simulink library "mlepLibrary"  (R2018a)
settings: Solver=ode45  StartTime=0.0  StopTime=10.0  RelTol=1e-3
undefined symbols (not defined in the file or in its folder): cs_val, mlepBlk_callback
settings Model: Creator=willyg  LastModifiedBy=E592090
settings DataIOCC: LimitDataPoints=on  SaveFormat=Array  SignalLoggingSaveFormat=ModelDataLogs
settings OptimizationCC: BlockReduction=off  BooleanDataType=off  LifeSpan=inf
settings DebuggingCC: SaveWithParameterizedLinksMsg=none  UnderspecifiedInitializationDetection=Classic  MergeDetectMultiDrivingBlocksExec=none  SignalResolutionControl=TryResolveAllWithWarning  MultiTaskDSMMsg=warning  MultiTaskCondExecSysMsg=none  SFUnexpectedBacktrackingDiag=warning  SFNoUnconditionalDefaultTransitionDiag=warning  SFExecutionAtInitializationDiag=none
settings HardwareCC: ProdBitPerPointer=32  ProdBitPerSizeT=32  ProdBitPerPtrDiffT=32  ProdLargestAtomicFloat=None  ProdIntDivRoundTo=Undefined  ProdEndianess=Unspecified  ProdWordSize=32  ProdHWDeviceType=32-bit Generic  TargetUnknown=on
settings ModelReferenceCC: PropagateSignalLabelsOutOfModel=off
settings CodeAppCC: StateflowObjectComments=on
settings GRTTargetCC: TargetLangStandard=C89/C90 (ANSI)  GeneratePreprocessorConditionals=Disable all
settings ConfigComp: CovMetricSettings=dw  CovHtmlReporting=on  CovSaveCumulativeToWorkspaceVar=on  CovSaveSingleToWorkspaceVar=on  CovExternalEMLEnable=off

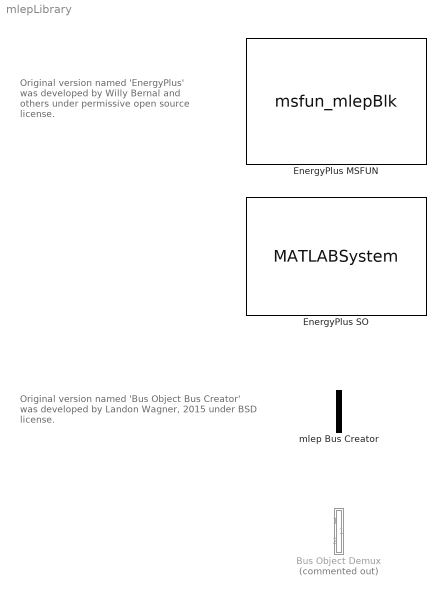
== system mlepLibrary ==
  note: Original version named 'EnergyPlus'
      | was developed by Willy Bernal and
      | others under permissive open source
      | license.
  note: Original version named 'Bus Object Bus Creator'
      | was developed by Landon Wagner, 2015 under
      | BSD license.
  Bus Object Demux : Subsystem  Commented=on  mask{busType=Bus: epInbus, bs_done=[]}
      mask prompts: busType "Bus Type"
      mask TypeOptions busType: Bus: epInbus | Bus: epOutbus
      mask Callback busType:
      | % Using variable names terminated with "_BOBC" to lessen the chances of
      | % collisions with existing workspace variables.
      | 
      | % Get the current block handle and mask handle.
      | handleCreator_BOBC = gcbh;
      | maskObj_BOBC       = Simulink.Mask.get(gcb);
      | 
      | % Get a list of variables in the workspace in order to search for the '1x1
      | % Bus' types.
      | wsVars_BOBC = whos;
      | 
      | % Reset the 'TypeOptions' bus list in case some '1x1 Bus' types have been
      | % deleted from or added to the workspace.
      | opts = {'<empty>'};
      | 
      | % Current number of options
      | old_opts = maskObj_BOBC.Parameters.TypeOptions;
      | 
      | % Reset the bus count.
      | busCount_BOBC = 0;
      | 
      | for index_BOBC = 1:length(wsVars_BOBC)
      | 
      |    % If the variable is a bus object...
      |    if strcmp(wsVars_BOBC(index_BOBC).class, 'Simulink.Bus')
      | 
      |       busCount_BOBC = busCount_BOBC + 1;
      | 
      |       % ... add it to the TypeOptions of the mask.
      |       opts(busCount_BOBC) = {['Bus: ', wsVars_BOBC(index_BOBC).name]};
      |    end
      | end
      | 
      | if busCount_BOBC == 0
      | 
      |    % If there are NO bus objects in the workspace then provide a warning
      |    % popup...
      |    %warning('There are currently no bus objects in the workspace - you have no use for this block. Use a normal Bus Creator instead.')
      | 
      |    % ... and do nothing.
      | % elseif ~strcmp(get_param(handleCreator_BOBC, 'OutDataTypeStr'), 'Inherit: auto')
      | %
      | %    % If the currently selected bus data type ('OutDataTypeStr') is not
      | %    % 'Inherit: auto' (i.e., if we are reopening the mask.) then get the
      | %    % current 'OutDataTypeStr' and 'maskVal.' ('maskVal' is the selected
      | %    % 'TypeOptions' list member.)
      | %    outDatStr_BOBC = get_param(handleCreator_BOBC, 'OutDataTypeStr');
      | %    maskVal_BOBC   = get_param(handleCreator_BOBC, 'MaskValues');
      | %
      | %    if ~strcmp(outDatStr_BOBC, maskVal_BOBC{1})
      | %
      | %       % Upon re-opening the mask if the default 'TypeOptions' list member
      | %       % (The first one.) contained in 'maskVal' does not match the
      | %       % currently selected bus data type ('OutDataTypeStr') then set the
      | %       % 'TypeOptions' list member to the selected bus data type. (Cuts down
      | %       % on confusion to have the displayed list member match the selected
      | %       % bus data type rather than the first entry.)
      | %       set_param(handleCreator_BOBC, 'MaskValues', {outDatStr_BOBC});
      | %    end
      | end
      | 
      | if ~strcmp([old_opts{:}],[opts{:}])
      |     maskObj_BOBC.Parameters.TypeOptions = opts;
      | end
      | 
      | % Clean up the workspace.
      | clear  handleCreator_BOBC  maskObj_BOBC     wsVars_BOBC ...
      |             busCount_BOBC    index_BOBC  outDatStr_BOBC ...
      |              maskVal_BOBC          opts        old_opts
      mask DialogControl applyMOCBSelection Prompt: Select signals
      mask DialogControl applyMOCBSelection Callback: run('clbk.m');
  EnergyPlus MSFUN : M-S-Function  InitFcn=mlepBlk_callback(gcb,'InitFcn');  FunctionName=msfun_mlepBlk  Parameters=work_dir, rel_path, fname, weather_profile, nout, timeout, eplus_path, bcvtb_dir, port, host  mask(EnergyPlus Cosimulation){work_dir=, rel_path=on, fname=idf_file, weather_profile=USA_IL_Chicago-OHare.Intl.AP.725300_TMY3, time_step=900, nout=2, timeout=10, mlep_defaults=on, eplus_path=, bcvtb_dir=, port=0, host=}
      mask prompts: work_dir "MLE+ working directory (empty = current directory)"; rel_path "Relative path"; fname "IDF file name"; weather_profile "EnergyPlus weather profile"; time_step "Time step (s)"; nout "Number of real outputs"; timeout "Communication timeout (s)"; mlep_defaults "Use default MLE+ settings"; eplus_path "EnergyPlus executable path (empty = default)"; bcvtb_dir "BCVTB directory (empty = default)"; port "Socket port (0 = auto)"; host "Socket host (empty = localhost)"
      mask help: This block implements cosimulation with EnergyPlus by allowing Simulink to exchange input and output data with it. Currently, EnergyPlus only supports real data.
      settings: PreSaveFcn=mlepBlk_callback(gcb,'PreSaveFcn');
      mask Help:
      | Simulate a building model using EnergyPlus
      | 
      | <h2>Description</h2>
      | This block implements <a href="http://apps1.eere.energy.gov/buildings/energyplus/">EnergyPlus</a> cosimulation by allowing Simulink to exchange input and output data with EnergyPlus at each time step.
      | 
      | When a simulation starts, this block starts EnergyPlus in parallel. During simulation, EnergyPlus exchanges data with Simulink using the <a href="http://simulationresearch.lbl.gov/bcvtb">Building Controls Virtual Test Bed</a> (BCVTB) interface via <a href="http://mlab.seas.upenn.edu/mlep/">MLE+</a>.
      | 
      | Detailed information about the interface is available in the MLE+ manual.
      | 
      | <h2>Requirements</h2>
      | Requires <a href="http://apps1.eere.energy.gov/buildings/energyplus/">EnergyPlus</a> and <a href="http://mlab.seas.upenn.edu/mlep/">MLE+</a>. In addition, requires a properly configured EnergyPlus model file (IDF) and BCVTB configuration file; see Comments.
      | 
      | <h2>Input</h2>
      | Block input <b>input</b> is a real-valued vector of EnergyPlus inputs corresponding to the inputs listed in the BCVTB config file <code>variables.cfg</code> (in order).
      | 
      | <h2>Output</h2>
      | The block outputs are, in order:
      | <dl>
      |   <dt><b>flag</b></dt><dd>Status flag for EnergyPlus: 0 if OK, non-zero for error</dd>
      |   <dt><b>time</b></dt><dd>Current simulation time of EnergyPlus (s)</dd>
      |   <dt><b>output</b></dt><dd>Real-valued vector of EnergyPlus outputs corresponding to the outputs listed in the BCVTB config file <code>variables.cfg</code> (in order).</dd>
      | </dl>
      | 
      | <h2>Parameters</h2>
      | The block mask provides inputs for all required MLE+ configuration parameters. The mask includes two tabs. The <i>Model</i> tab provides information about the EnergyPlus model to run, and the <i>MLE+</i> provides inputs for MLE+ settings.
      | 
      | String inputs in the block mask, such as paths and file names, are not evaluated prior to passing to MLE+. Therefore, MATLAB expressions which evaluate to strings (for example, <code>[pwd '/somedir']</code>) may not be passed directly. Instead, use an initialization script to evaluate these expressions and store the evaluated strings in the block mask prior to running the simulation.
      | 
      | <h3>Model Tab</h3>
      | The <i>Model</i> tab provides inputs for the following parameters:
      | <dl>
      |   <dt><b>MLE+ working directory</b></dt>
      |     <dd>The MLE+ and EnergyPlus working directory. <i>EnergyPlus will read from and write to this directory.</i></dd>
      |   <dt><b>Relative path</b></dt>
      |     <dd>Check this box if <b>MLE+ working directory</b> is specified relative to the current MATLAB working directory. <i>Otherwise, the block will treat <b>MLE+ working directory</b> as an absolute path.</i></dd>
      |   <dt><b>IDF file name</b></dt>
      |     <dd>The EnergyPlus model file (IDF), with or without the <code>.idf</code> extension. <i>This file must be included in the <b>MLE+ working directory</b>. Do not specify an absolute path for this file!</i></dd>
      |   <dt><b>EnergyPlus weather profile</b></dt>
      |     <dd>The EnergyPlus weather file (EPW), with or without the <code>.epw</code> extension. <i>A matching weather file must be included in your EnergyPlus installation's <code>WeatherData</code> directory.</i></dd>
      |   <dt><b>Time Step</b></dt>
      |     <dd>The EnergyPlus time step (s). <i>This need not be the same as the Simulink time step.</i></dd>
      |   <dt><b>Number of Real Outputs</b></dt>
      |     <dd>The number of real outputs from EnergyPlus. <i>This number must match the number of output variables in <code>variables.cfg</code>.</i></dd>
      | </dl>
      | 
      | <h3>MLE+ Tab</h3>
      | The <i>MLE+</i> tab provides inputs for the following parameters:
      | <dl>
      |   <dt><b>Communication timeout</b></dt>
      |     <dd>Time delay (s) before communication between MLE+ and EnergyPlus times out.</dd>
      |   <dt><b>Use default MLE+ settings</b></dt>
      |     <dd>Uncheck this box to gain access to the remaining settings in the <i>MLE+</i> tab.</dd>
      |   <dt><b>EnergyPlus executable path</b></dt>
      |     <dd>The full path to the EnergyPlus executable (e.g. <code>C:\EnergyPlusV8-1-0\RunEPlus.bat</code>); leave blank to use default MLE+ setting.</dd>
      |   <dt><b>BCVTB directory</b></dt>
      |     <dd>The full path to the directory where the BCVTB library resides; leave blank to use default MLE+ setting.</dd>
      |   <dt><b>Socket port</b></dt>
      |     <dd>The port to use for communication with EnergyPlus; enter <code>0</code> to allow MLE+ to automatically select a port.</dd>
      |   <dt><b>Socket host</b></dt>
      |     <dd>The IP address of the host machine where EnergyPlus runs; leave blank to use localhost (the local computer).</dd>
      | </dl>
      | 
      | <h2>Comments</h2>
      | <ol>
      |   <li>For fixed time step simulation in Simulink, the EnergyPlus time step must be an exact multiple of the Simulink time step.</li>
      |   <li>Summary of requirements for EnergyPlus model file (<code>*.idf</code>):
      |     <ol type="a">
      | 	  <li>The EnergyPlus time step specified in the file must match the value specified in the block mask.</li>
      | 	  <li>The start date and time in EnergyPlus must correspond to the start time of the Simulink simulation (usually <i>t</i> = 0 s).</li>
      | 	  <li>The <i>ExternalInterface</i> object must be defined and assigned the name  <code>PtolemyServer</code>.</li>
      | 	  <li>The file must include <i>ExternalInterface</i> definitions all inputs specified in the BCVTB config file, and the names must match.</li>
      | 	  <li>The file must include <i>Output</i> definitions all outputs specified in the BCVTB config file, and the names must match.</li>
      | 	</ol>
      |   </li>
      |   <li>Summary of requirements for BCVTB config file (<code>variables.cfg</code>):
      |     <ol type="a">
      | 	  <li>The file be located in the MLE+ working directory specified in the block mask.</li>
      | 	  <li>Number of output variables must match the value specified in the block mask.</li>
      | 	  <li>Order of input variables must match the order of elements in the input vector in Simulink.</li>
      | 	  <li>Order of output variables must match the order of elements in the output vector in Simulink.</li>
      | 	</ol>
      |   <li>For more details regarding the implementation of MLE+, the meaning of the parameters, and creating the BCVTB configuration file, see the MLE+ <a href="http://mlab.seas.upenn.edu/mlep/">documentation</a>.</li>
      | </ol>
      | 
      | <h2>References</h2>
      | <ol>
      |   <li>W. Bernal, M. Behl, T. X. Nghiem, and R. Mangharam, "MLE+: A Tool for Integrated Design and Deployment of Energy Efficient Building Controls," 4th ACM Workshop On Embedded Sensing Systems For Energy-Efficiency In Buildings, (BuildSys '12), Toronto, Canada, 2012. Available: <a href="http://repository.upenn.edu/mlab_papers/51/">http://repository.upenn.edu/mlab_papers/51/</a></li>
      | </ol>
      mask Callback mlep_defaults: mlepBlk_callback(gcb, 'MaskConfig');
      mask DialogControl ParameterTabVar0 Prompt: Model
      mask DialogControl ParameterTabVar01 Prompt: MLE+
      mask Display:
      | image(imread('mlepBlkIcon.jpg'))
      | 
      | text(0.05,.1,'EnergyPlus\nCo-simulation');
      | % Inputs
      | c = 0.80*[1 1 1];
      | x = [0 1 1 0 0];
      | y = [0 0 1 1 0];
      | h = 0.09;
      | 
      | %color('white');
      | % x0 = 0;
      | % y0 = 0.448;
      | % w = 0.18;
      | % patch(x0 + w*x, y0 + h*y, c);
      | port_label('input', 1, 'Inputs');
      | 
      | % % Outputs
      | % w = 0.128;
      | % x0 = 1-w;
      | % y0 = 0.768;
      | % patch(x0 + w*x, y0 + h*y, c);
      | port_label('output', 1, 'Flag');
      | 
      | % w = 0.139;
      | % x0 = 1-w;
      | % y0 = 0.455;
      | % patch(x0 + w*x, y0 + h*y, c);
      | port_label('output', 2, 'Time');
      | 
      | % w = 0.215;
      | % x0 = 1-w;
      | % y0 = 0.13;
      | % patch(x0 + w*x, y0 + h*y, c);
      | port_label('output', 3, 'Outputs');
  EnergyPlus SO : MATLABSystem  System=so_mlepBlk  idfFile=in.idf  epwFile=in.epw  SimulateUsing=Code generation  useBus=on  inputBusName=epInbus  outputBusName=epOutbus
      mask Type: mlepSO
      mask Display:
      | image('mlepBlkIcon.jpg');
      | port_label('input',1,'epInbus');
      | port_label('output',1,'Flag');
      | port_label('output',2,'Time');
      | port_label('output',3,'epOutbus');
  mlep Bus Creator : BusCreator  Inputs=1  mask(BUS OBJECT Bus Creator){busType=Bus: epInbus}
      mask prompts: busType "Bus Type"
      mask help:
      | Provides users the cabability to painlessly, instantly customize bus creators of output data type 'Bus:' by selecting the bus object type from a drop down menu dynamically populated by bus objects in the workspace.
      |
      | After pressing the "Apply Selection" button signal lines into the creator are populated and named with the elements in the chosen bus saving the user from having to recall and fill out signal line names.
      |
      | NOTE that when copying a Bus Object Bus Creator from your locked Library the link to the Library is automatically broken. This saves the user from having to Unlock Links To Library (From the Library menu.), Disable Link and finally Break Link (Both from the Model menu.) for every placed instance of the block.
      settings: AttributesFormatString=%<OutDataTypeStr>  CopyFcn=set_param(gcb, 'LinkStatus', 'none')
      mask TypeOptions busType: Bus: epInbus | Bus: epOutbus
      mask Callback busType:
      | % Using variable names terminated with "_BOBC" to lessen the chances of
      | % collisions with existing workspace variables.
      | 
      | % Get the current block handle and mask handle.
      | handleCreator_BOBC = gcbh;
      | maskObj_BOBC       = Simulink.Mask.get(gcb);
      | 
      | % Get a list of variables in the workspace in order to search for the '1x1
      | % Bus' types.
      | wsVars_BOBC = whos;
      | 
      | % Reset the 'TypeOptions' bus list in case some '1x1 Bus' types have been
      | % deleted from or added to the workspace.
      | opts = {'<empty>'};
      | 
      | % Current number of options
      | old_opts = maskObj_BOBC.Parameters.TypeOptions;
      | 
      | % Reset the bus count.
      | busCount_BOBC = 0;
      | 
      | for index_BOBC = 1:length(wsVars_BOBC)
      | 
      |    % If the variable is a bus object...
      |    if strcmp(wsVars_BOBC(index_BOBC).class, 'Simulink.Bus')
      | 
      |       busCount_BOBC = busCount_BOBC + 1;
      | 
      |       % ... add it to the TypeOptions of the mask.
      |       opts(busCount_BOBC) = {['Bus: ', wsVars_BOBC(index_BOBC).name]};
      |    end
      | end
      | 
      | if busCount_BOBC == 0
      | 
      |    % If there are NO bus objects in the workspace then provide a warning
      |    % popup...
      |    warning('There are currently no bus objects in the workspace - you have no use for this block. Use a normal Bus Creator instead.')
      | 
      |    % ... and do nothing.
      | elseif ~strcmp(get_param(handleCreator_BOBC, 'OutDataTypeStr'), 'Inherit: auto')
      | 
      |    % If the currently selected bus data type ('OutDataTypeStr') is not
      |    % 'Inherit: auto' (i.e., if we are reopening the mask.) then get the
      |    % current 'OutDataTypeStr' and 'maskVal.' ('maskVal' is the selected
      |    % 'TypeOptions' list member.)
      |    outDatStr_BOBC = get_param(handleCreator_BOBC, 'OutDataTypeStr');
      |    maskVal_BOBC   = get_param(handleCreator_BOBC, 'MaskValues');
      | 
      |    if ~strcmp(outDatStr_BOBC, maskVal_BOBC{1})
      | 
      |       % Upon re-opening the mask if the default 'TypeOptions' list member
      |       % (The first one.) contained in 'maskVal' does not match the
      |       % currently selected bus data type ('OutDataTypeStr') then set the
      |       % 'TypeOptions' list member to the selected bus data type. (Cuts down
      |       % on confusion to have the displayed list member match the selected
      |       % bus data type rather than the first entry.)
      |       set_param(handleCreator_BOBC, 'MaskValues', {outDatStr_BOBC});
      |    end
      | end
      | 
      | if ~strcmp([old_opts{:}],[opts{:}])
      |     maskObj_BOBC.Parameters.TypeOptions = opts;
      | end
      | 
      | % Clean up the workspace.
      | clear  handleCreator_BOBC  maskObj_BOBC     wsVars_BOBC ...
      |             busCount_BOBC    index_BOBC  outDatStr_BOBC ...
      |              maskVal_BOBC          opts        old_opts
      mask DialogControl applyMOCBSelection Prompt: Apply Selection
      mask DialogControl applyMOCBSelection Callback:
      | % Using variable names terminated with "_BOBC" to lessen the chances of
      | % collisions with existing workspace variables.
      | 
      | % Get the current block, current block handle and mask handle.
      | currentBlock_BOBC  = gcb;
      | handleCreator_BOBC = gcbh;
      | 
      | % Get the desired bus type...
      | desiredBusType_BOBC = get_param(handleCreator_BOBC, 'busType');
      | 
      | % ... and set the 'OutDataTypeStr' to it.
      | set_param(handleCreator_BOBC, 'OutDataTypeStr', desiredBusType_BOBC);
      | 
      | %% First delete any existing lines on the port.
      | % Get the line handles.
      | lh_BOBC = get_param(handleCreator_BOBC, 'LineHandles');
      | 
      | % If any lines exist (Non- -1 line handles.), delete them and start over.
      | if max(lh_BOBC.Inport > 0)
      | 
      |    for index_BOBC = 1:length(lh_BOBC.Inport)
      | 
      |       if lh_BOBC.Inport(index_BOBC) > 0
      | 
      |          delete_line(lh_BOBC.Inport(index_BOBC))
      |       end
      |    end
      | end
      | 
      | %% Then work on adding new lines.
      | 
      | % Get the block path for 'add_line' function.
      | blockPath_BOBC = get_param(handleCreator_BOBC, 'Parent');
      | 
      | % Get the newly selected bus type ('OutDataTypeStr')...
      | mocbBusType_BOBC = get_param(currentBlock_BOBC, 'OutDataTypeStr');
      | 
      | % ... and parse off "Bus: " so the string of the desired bus contained in
      | % 'OutDataTypeStr' matches the raw workspace bus names.
      | mocbBusType_BOBC = mocbBusType_BOBC(6:end);
      | 
      | % Then evaluate the string containing the workspace bus name which will
      | % load the desired bus parameters.
      | busParams_BOBC = eval(mocbBusType_BOBC);
      | 
      | % From the parameters grab the number of lines to add.
      | numLines_BOBC = length(busParams_BOBC.Elements);
      | 
      | % Set the number of inputs of the masked bus creator to the number of lines
      | % to add.
      | set_param(handleCreator_BOBC, 'Inputs', num2str(numLines_BOBC));
      | 
      | % Set heigh
      | sz = get_param(handleCreator_BOBC, 'Position');
      | y0 = sz(2) + (sz(4)-sz(2))/2; % vertical center
      | h  = max(sz(4)-sz(2), numLines_BOBC*10); % height
      | sz = [sz(1), ...
      |       y0 - h/2, ...
      |       sz(3), ...
      |       y0 + h/2];
      | set_param(handleCreator_BOBC, 'Position', sz);
      | clear y0 h sz
      | 
      | % Get (Inputs.) port handles so we can grab the positions of them.
      | ph_BOBC = get_param(handleCreator_BOBC, 'PortHandles');
      | 
      | % Get longest signal name to adjust the line lenght right
      | names_BOBC = {busParams_BOBC.Elements.Name};
      | 
      | for index_BOBC = 1:numLines_BOBC
      | 
      |    % Get the position of input port number 'index_BOBC'.
      |    portPos_BOBC = get_param(ph_BOBC.Inport(index_BOBC), 'Position');
      | 
      |    % Add a line from 50 pixels left of the port position to the port
      |    % position. (This must be done because it's the lines that get named,
      |    % not the port positions.)
      |    portLine_BOBC = add_line(blockPath_BOBC, ...
      |        [portPos_BOBC - [ceil(50/10/2*max(strlength(names_BOBC)))+10 0]; portPos_BOBC]);
      | 
      |    % Rename the new line to the bus 'index_BOBC-st/nd/rd/th' element name.
      |    set_param(portLine_BOBC, 'Name', busParams_BOBC.Elements(index_BOBC).Name)
      | end
      | 
      | %% Cleanup the workspace.
      | clear    currentBlock_BOBC  handleCreator_BOBC      index_BOBC ...
      |        desiredBusType_BOBC             lh_BOBC  blockPath_BOBC ...
      |           mocbBusType_BOBC      busParams_BOBC   numLines_BOBC ...
      |                    ph_BOBC        portPos_BOBC   portLine_BOBC ...
      |                 names_BOBC

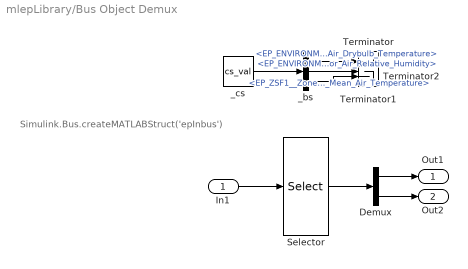
== system mlepLibrary/Bus Object Demux ==
  note: Simulink.Bus.createMATLABStruct('epInbus')
  In1 : Inport
  Demux : Demux  Outputs=2
  Selector : Selector  InputPortWidth=12  IndexOptions=Index vector (dialog)  Indices=[1 2]  OutputSizes=1
  Terminator : Terminator
  Terminator1 : Terminator
  Terminator2 : Terminator
  _bs : BusSelector  OutputSignals=EP_ENVIRONMENT__Site_Outdoor_Air_Drybulb_Temperature,EP_ENVIRONMENT__Site_Outdoor_Air_Relative_Humidity,EP_ZSF1__Zone_Mean_Air_Temperature
      mask init:
      | maskObj = Simulink.Mask.get(get_param(gcb,'Parent'));
      | maskObj.Initialization = '';
  _cs : Constant  Value=cs_val  OutDataTypeStr=Bus: epOutbus
  Out1 : Outport
  Out2 : Outport  Port=2
  wires:
  _cs/1 -> _bs/1
  In1/1 -> Selector/1
  Selector/1 -> Demux/1
  Demux/1 -> Out1/1
  Demux/2 -> Out2/1
  _bs/1 -> Terminator/1  "<EP_ENVIRONMENT__Site_Outdoor_Air_Drybulb_Temperature>"
  _bs/2 -> Terminator1/1  "<EP_ENVIRONMENT__Site_Outdoor_Air_Relative_Humidity>"
  _bs/3 -> Terminator2/1  "<EP_ZSF1__Zone_Mean_Air_Temperature>"
